simulink model "lab01_1"  (Simulink 9.2)
settings: Solver=ode45  StartTime=0.0  StopTime=10.0  RelTol=1e-3  EnableMultiTasking=on
settings Model: Creator=murad  LastModifiedBy=murad
settings DataIOCC: SignalLoggingName=sigsOut
settings OptimizationCC: LifeSpan=auto
settings DebuggingCC: SaveWithParameterizedLinksMsg=none  SignalResolutionControl=TryResolveAllWithWarning  MultiTaskDSMMsg=warning  MultiTaskCondExecSysMsg=none  FcnCallInpInsideContextMsg=error  StateNameClashWarn=none  SFUnexpectedBacktrackingDiag=error  SFNoUnconditionalDefaultTransitionDiag=error  SFExecutionAtInitializationDiag=warning
settings HardwareCC: TargetUnknown=on
settings SFSimCC: SimUseLocalCustomCode=on
settings RTWCC: RTWUseLocalCustomCode=on
settings CodeAppCC: StateflowObjectComments=off
settings GRTTargetCC: TargetLangStandard=C99 (ISO)  GeneratePreprocessorConditionals=Use local settings
settings ConfigComp: CovExternalEMLEnable=on

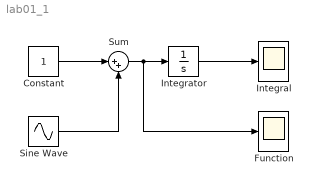
== system lab01_1 ==
  Constant : Constant
  Function : Scope
  Integral : Scope
  Integrator : Integrator
  Sine Wave : Sin  SampleTime=0
  Sum : Sum  Inputs=|++  SaturateOnIntegerOverflow=on
  wires:
  Constant/1 -> Sum/1
  Sum/1 -> Function/1, Integrator/1
  Integrator/1 -> Integral/1
  Sine Wave/1 -> Sum/2
